simulink model "gm_broadwayIPC_2024b"  (R2024b)
settings: Solver=FixedStepDiscrete  StartTime=0.0  StopTime=2  RelTol=1e-3
undefined symbols (not defined in the file or in its folder): gray
libraries: hdlsllib x28, visionhdlio x6, visionsources x2
Description:
  | Sobel Edge Detection Using the MATLAB(R) Function Block
  | This example shows how to use HDL Coder(TM) to check,
  | generate, and verify HDL code for a Sobel Edge Detection
  | block built using the MATLAB Function block.
settings Model: Creator=The MathWorks, Inc.  LastModifiedBy=Chris
settings SolverCC: AlgebraicLoopSolver=TrustRegion
settings DataIOCC: LimitDataPoints=on  SaveFormat=Array  SignalLogging=off  ReturnWorkspaceOutputs=off
settings OptimizationCC: BlockReduction=off  ConditionallyExecuteInputs=off  DefaultParameterBehavior=Inlined  ExpressionDepthLimit=2147483647  InitFltsAndDblsToZero=on  EfficientMapNaN2IntZero=off  LifeSpan=inf
settings DebuggingCC: AlgebraicLoopMsg=error  SaveWithParameterizedLinksMsg=none  UnderspecifiedInitializationDetection=Classic  MergeDetectMultiDrivingBlocksExec=none  SignalResolutionControl=TryResolveAllWithWarning  InheritedTsInSrcMsg=none  MultiTaskDSMMsg=warning  MultiTaskCondExecSysMsg=none  SingleTaskRateTransMsg=error  IntegerOverflowMsg=none  ParameterPrecisionLossMsg=none  FcnCallInpInsideContextMsg=warning  UnconnectedInputMsg=warning  UnconnectedOutputMsg=warning  UnconnectedLineMsg=warning  AllowSymbolicDim=off  StateNameClashWarn=warning  StrictBusMsg=ErrorOnBusTreatedAsVector  SFUnexpectedBacktrackingDiag=warning  SFNoUnconditionalDefaultTransitionDiag=warning  SFExecutionAtInitializationDiag=none  IntegerSaturationMsg=none  ArithmeticOperatorsInVariantConditions=warning
settings HardwareCC: ProdBitPerPointer=32  ProdBitPerSizeT=32  ProdBitPerPtrDiffT=32  ProdLargestAtomicFloat=None  ProdIntDivRoundTo=Undefined  ProdEndianess=Unspecified  ProdWordSize=32  ProdHWDeviceType=ASIC/FPGA  TargetHWDeviceType=32-bit Generic  ProdEqTarget=off
settings ModelReferenceCC: EnableRefExpFcnMdlSchedulingChecks=on  PropagateSignalLabelsOutOfModel=off
settings SFSimCC: SimUseLocalCustomCode=off  CustomCodeUndefinedFunction=UseInterfaceOnly
settings RTWCC: RTWUseLocalCustomCode=off  GPUComputeCapability=3.5  DLArmComputeVersion=19.05
settings CodeAppCC: StateflowObjectComments=on
settings GRTTargetCC: TargetFcnLib=ansi_tfl_tmw.mat  TargetLangStandard=C89/C90 (ANSI)  CombineOutputUpdateFcns=off  GRTInterface=on
settings ConfigComp: CovMetricSettings=dw  CovSaveCumulativeToWorkspaceVar=on  CovSaveSingleToWorkspaceVar=on  CovExternalEMLEnable=off

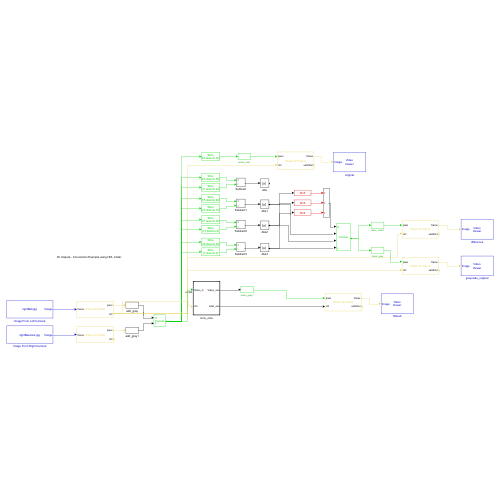
[thumbnail: Simulink's stored preview of the top-level diagram]
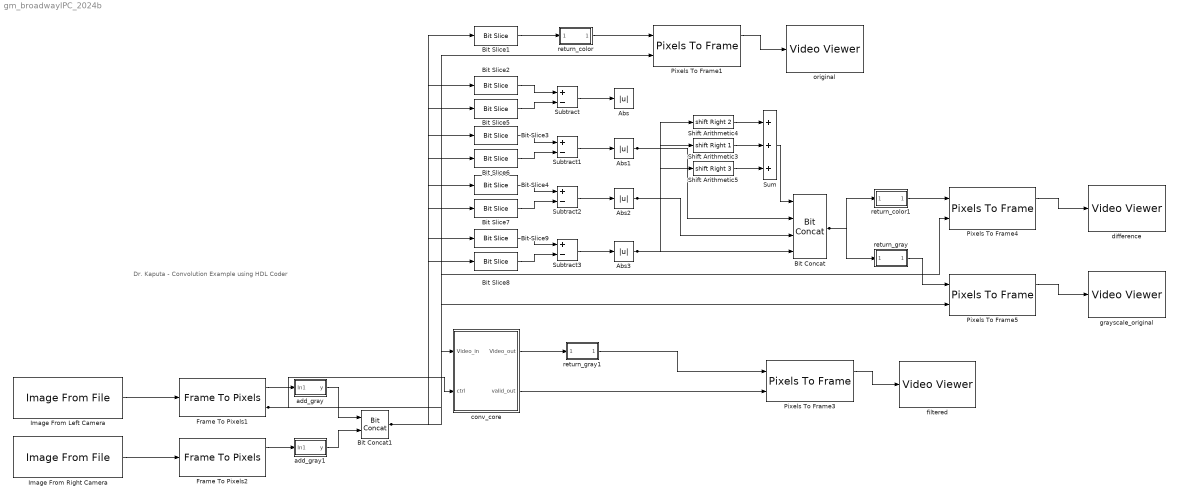
== system gm_broadwayIPC_2024b ==
  note: Dr. Kaputa - Convolution Example using HDL Coder
  Abs{,1..3} (4 alike) : Abs  OutDataTypeStr=uint8
  Bit Concat : hdlsllib/Logic and Bit Operations/Bit Concat  numInputs=4
  Bit Concat1 : hdlsllib/Logic and Bit Operations/Bit Concat  numInputs=2
  Bit Slice1 : hdlsllib/Logic and Bit Operations/Bit Slice  lidx=63  ridx=32
  Bit Slice2 : hdlsllib/Logic and Bit Operations/Bit Slice  lidx=63  ridx=56
  Bit Slice3 : hdlsllib/Logic and Bit Operations/Bit Slice  lidx=55  ridx=48
  Bit Slice4 : hdlsllib/Logic and Bit Operations/Bit Slice  lidx=47  ridx=40
  Bit Slice5 : hdlsllib/Logic and Bit Operations/Bit Slice  lidx=31  ridx=24
  Bit Slice6 : hdlsllib/Logic and Bit Operations/Bit Slice  lidx=23  ridx=16
  Bit Slice7 : hdlsllib/Logic and Bit Operations/Bit Slice  lidx=15  ridx=8
  Bit Slice8 : hdlsllib/Logic and Bit Operations/Bit Slice  lidx=7  ridx=0
  Bit Slice9 : hdlsllib/Logic and Bit Operations/Bit Slice  lidx=39  ridx=32
  Frame To Pixels1 : visionhdlio/Frame To Pixels  NumComponents=3  NumPixels=1  VideoFormat=Custom  ActivePixelsPerLine=R  ActiveVideoLines=C  TotalPixelsPerLine=R  TotalVideoLines=C  StartingActiveLine=1  FrontPorch=0  SampleTime=0  VideoFormatCache=Custom  ActivePixelsPerLineCache=R  ActiveVideoLinesCache=C  TotalPixelsPerLineCache=R  TotalVideoLinesCache=C  StartingActiveLineCache=1  FrontPorchCache=0
  Frame To Pixels2 : visionhdlio/Frame To Pixels  NumComponents=3  NumPixels=1  VideoFormat=Custom  ActivePixelsPerLine=R  ActiveVideoLines=C  TotalPixelsPerLine=R  TotalVideoLines=C  StartingActiveLine=1  FrontPorch=0  SampleTime=0  VideoFormatCache=Custom  ActivePixelsPerLineCache=R  ActiveVideoLinesCache=C  TotalPixelsPerLineCache=R  TotalVideoLinesCache=C  StartingActiveLineCache=1  FrontPorchCache=0
  Image From Left Camera : visionsources/Image From File  Tag=vipblks_nd  FileName=C:\Users\Chris\Documents\Repos\WiiSports\TennisTracker\BoradwaySimulink\rightBall.jpg  Ts=1  imagePorts=One multidimensional signal  OutPortLabels=R|G|B  ImageDataType=Inherit from input image  sdImageDataType=uint(8)  Signed=on  WordLength=16  FractionLengthMode=User-defined  FractionLength=15
  Image From Right Camera : visionsources/Image From File  Tag=vipblks_nd  FileName=C:\Users\Chris\Documents\Repos\WiiSports\TennisTracker\BoradwaySimulink\rightBaseline.jpg  Ts=1  imagePorts=One multidimensional signal  OutPortLabels=R|G|B  ImageDataType=Inherit from input image  sdImageDataType=uint(8)  Signed=on  WordLength=16  FractionLengthMode=User-defined  FractionLength=15
  Pixels To Frame1 : visionhdlio/Pixels To Frame  NumComponents=3  NumPixels=1  VideoFormat=Custom  ActivePixelsPerLine=R  ActiveVideoLines=C  TotalPixelsPerLine=R  TotalVideoLines=C  VideoFormatCache=Custom  ActivePixelsPerLineCache=R  ActiveVideoLinesCache=C  TotalPixelsPerLineCache=R  TotalVideoLinesCache=C
  Pixels To Frame3 : visionhdlio/Pixels To Frame  NumComponents=1  NumPixels=1  VideoFormat=Custom  ActivePixelsPerLine=R  ActiveVideoLines=C  TotalPixelsPerLine=R  TotalVideoLines=C  VideoFormatCache=Custom  ActivePixelsPerLineCache=R  ActiveVideoLinesCache=C  TotalPixelsPerLineCache=R  TotalVideoLinesCache=C
  Pixels To Frame4 : visionhdlio/Pixels To Frame  NumComponents=3  NumPixels=1  VideoFormat=Custom  ActivePixelsPerLine=R  ActiveVideoLines=C  TotalPixelsPerLine=R  TotalVideoLines=C  VideoFormatCache=Custom  ActivePixelsPerLineCache=R  ActiveVideoLinesCache=C  TotalPixelsPerLineCache=R  TotalVideoLinesCache=C
  Pixels To Frame5 : visionhdlio/Pixels To Frame  NumComponents=1  NumPixels=1  VideoFormat=Custom  ActivePixelsPerLine=R  ActiveVideoLines=C  TotalPixelsPerLine=R  TotalVideoLines=C  VideoFormatCache=Custom  ActivePixelsPerLineCache=R  ActiveVideoLinesCache=C  TotalPixelsPerLineCache=R  TotalVideoLinesCache=C
  Shift Arithmetic3 : ArithShift  BitShiftNumber=1  BitShiftDirection=Right
  Shift Arithmetic4 : ArithShift  BitShiftNumber=2  BitShiftDirection=Right
  Shift Arithmetic5 : ArithShift  BitShiftNumber=3  BitShiftDirection=Right
  Subtract{,1..3} (4 alike) : Sum  Inputs=+-
  Sum : Sum  Inputs=+++  OutDataTypeStr=uint8
  add_gray : Subsystem
  add_gray1 : Subsystem
  conv_core : Subsystem  TreatAsAtomicUnit=on
  difference : VideoViewer  FigPos=[994 1078 927 429]
  filtered : VideoViewer  colormapValue=gray(256)  FigPos=[66 1078 927 429]
  grayscale_original : VideoViewer  FigPos=[65 538 927 429]
  original : VideoViewer  FigPos=[995 538 927 429]
  return_color : Subsystem
  return_color1 : Subsystem
  return_gray : Subsystem
  return_gray1 : Subsystem
  wires:
  return_gray1/1(RGBVector) -> Pixels To Frame3/1
  conv_core/1(Video_out) -> return_gray1/1(RGB)
  Bit Concat/1 -> return_color1/1(RGB), return_gray/1(RGB)
  Sum/1 -> Bit Concat/1
  Abs1/1 -> Bit Concat/2, Shift Arithmetic4/1
  Abs2/1 -> Bit Concat/3, Shift Arithmetic3/1
  Abs3/1 -> Bit Concat/4, Shift Arithmetic5/1
  Shift Arithmetic4/1 -> Sum/1
  Shift Arithmetic3/1 -> Sum/2
  Shift Arithmetic5/1 -> Sum/3
  return_gray/1(RGBVector) -> Pixels To Frame5/1
  Pixels To Frame5/1 -> grayscale_original/1
  Bit Slice8/1 -> Subtract3/2
  Bit Slice9/1 -> Subtract3/1
  Bit Slice7/1 -> Subtract2/2
  Bit Slice4/1 -> Subtract2/1
  Bit Slice6/1 -> Subtract1/2
  Bit Slice3/1 -> Subtract1/1
  Bit Slice5/1 -> Subtract/2
  Bit Slice2/1 -> Subtract/1
  Subtract3/1 -> Abs3/1
  Subtract2/1 -> Abs2/1
  Subtract1/1 -> Abs1/1
  return_color1/1(RGBVector) -> Pixels To Frame4/1
  Subtract/1 -> Abs/1
  Pixels To Frame4/1 -> difference/1
  Bit Slice1/1 -> return_color/1(RGB)
  add_gray1/1(y) -> Bit Concat1/2
  add_gray/1(y) -> Bit Concat1/1
  Frame To Pixels2/1 -> add_gray1/1(In1)
  Frame To Pixels1/2 -> conv_core/2(ctrl), Pixels To Frame4/2, Pixels To Frame5/2, Pixels To Frame1/2
  Image From Right Camera/1 -> Frame To Pixels2/1
  Bit Concat1/1 -> conv_core/1(Video_in), Bit Slice5/1, Bit Slice3/1, Bit Slice6/1, Bit Slice4/1, Bit Slice7/1, Bit Slice9/1, Bit Slice8/1, Bit Slice2/1, Bit Slice1/1
  conv_core/2(valid_out) -> Pixels To Frame3/2
  Pixels To Frame3/1 -> filtered/1
  Frame To Pixels1/1 -> add_gray/1(In1)
  return_color/1(RGBVector) -> Pixels To Frame1/1
  Pixels To Frame1/1 -> original/1
  Image From Left Camera/1 -> Frame To Pixels1/1

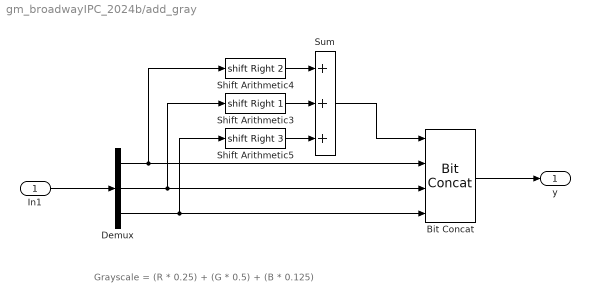
== system gm_broadwayIPC_2024b/add_gray ==
  note: Grayscale = (R * 0.25) + (G * 0.5) + (B * 0.125)
  In1 : Inport
  Bit Concat : hdlsllib/Logic and Bit Operations/Bit Concat  numInputs=4
  Demux : Demux  Outputs=3
  Shift Arithmetic3 : ArithShift  BitShiftNumber=1  BitShiftDirection=Right
  Shift Arithmetic4 : ArithShift  BitShiftNumber=2  BitShiftDirection=Right
  Shift Arithmetic5 : ArithShift  BitShiftNumber=3  BitShiftDirection=Right
  Sum : Sum  Inputs=+++  OutDataTypeStr=uint8
  y : Outport
  wires:
  Shift Arithmetic5/1 -> Sum/3
  Shift Arithmetic3/1 -> Sum/2
  Shift Arithmetic4/1 -> Sum/1
  Sum/1 -> Bit Concat/1
  Demux/3 -> Bit Concat/4, Shift Arithmetic5/1
  Demux/1 -> Bit Concat/2, Shift Arithmetic4/1
  Demux/2 -> Bit Concat/3, Shift Arithmetic3/1
  In1/1 -> Demux/1
  Bit Concat/1 -> y/1

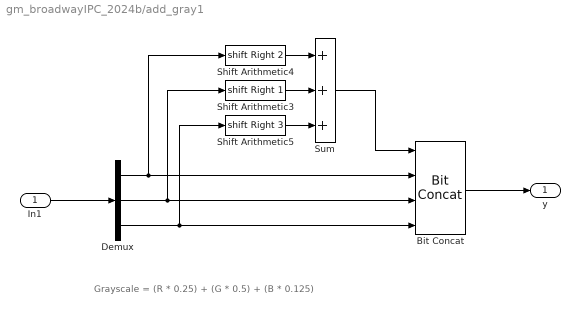
== system gm_broadwayIPC_2024b/add_gray1 ==
  note: Grayscale = (R * 0.25) + (G * 0.5) + (B * 0.125)
  In1 : Inport
  Bit Concat : hdlsllib/Logic and Bit Operations/Bit Concat  numInputs=4
  Demux : Demux  Outputs=3
  Shift Arithmetic3 : ArithShift  BitShiftNumber=1  BitShiftDirection=Right
  Shift Arithmetic4 : ArithShift  BitShiftNumber=2  BitShiftDirection=Right
  Shift Arithmetic5 : ArithShift  BitShiftNumber=3  BitShiftDirection=Right
  Sum : Sum  Inputs=+++  OutDataTypeStr=uint8
  y : Outport
  wires:
  Sum/1 -> Bit Concat/1
  Shift Arithmetic5/1 -> Sum/3
  Shift Arithmetic3/1 -> Sum/2
  Shift Arithmetic4/1 -> Sum/1
  Demux/3 -> Bit Concat/4, Shift Arithmetic5/1
  Demux/1 -> Bit Concat/2, Shift Arithmetic4/1
  Demux/2 -> Bit Concat/3, Shift Arithmetic3/1
  In1/1 -> Demux/1
  Bit Concat/1 -> y/1

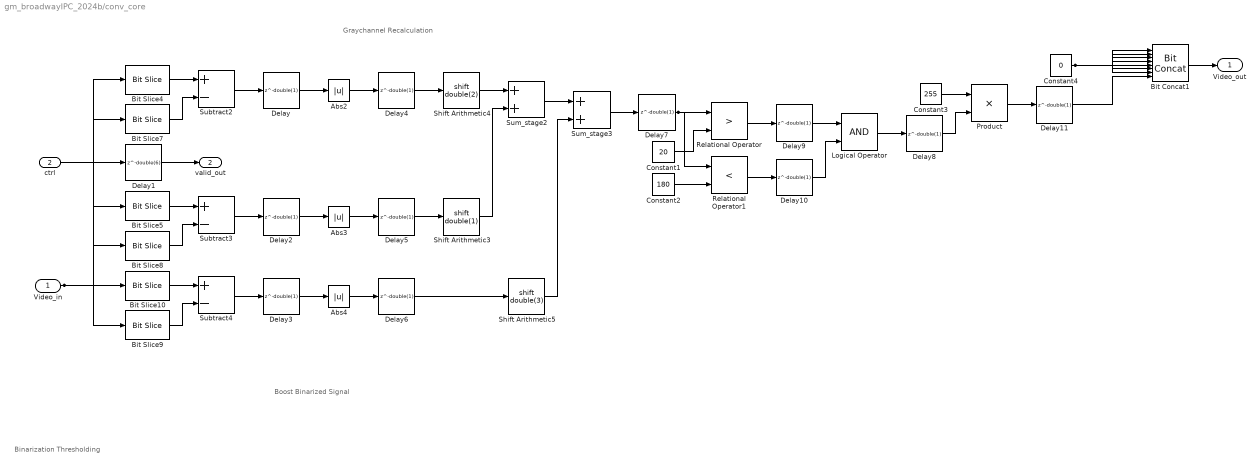
== system gm_broadwayIPC_2024b/conv_core ==
  note: Boost Binarized Signal
  note: Binarization Thresholding
  note: Graychannel Recalculation
  Video_in : Inport  OutDataTypeStr=fixdt(0, 64, 0)  PortDimensions=1  SampleTime=2.77039007092199e-06
  ctrl : Inport  Port=2
  Abs2 : Abs  SampleTime=2.77039007092199e-06  OutDataTypeStr=uint8  SaturateOnIntegerOverflow=off
  Abs3 : Abs  SampleTime=2.77039007092199e-06  OutDataTypeStr=uint8  SaturateOnIntegerOverflow=off
  Abs4 : Abs  SampleTime=2.77039007092199e-06  OutDataTypeStr=uint8  SaturateOnIntegerOverflow=off
  Bit Concat1 : hdlsllib/Logic and Bit Operations/Bit Concat  numInputs=8
  Bit Slice10 : hdlsllib/Logic and Bit Operations/Bit Slice  lidx=double(39)  ridx=double(32)
  Bit Slice4 : hdlsllib/Logic and Bit Operations/Bit Slice  lidx=double(55)  ridx=double(48)
  Bit Slice5 : hdlsllib/Logic and Bit Operations/Bit Slice  lidx=double(47)  ridx=double(40)
  Bit Slice7 : hdlsllib/Logic and Bit Operations/Bit Slice  lidx=double(23)  ridx=double(16)
  Bit Slice8 : hdlsllib/Logic and Bit Operations/Bit Slice  lidx=double(15)  ridx=double(8)
  Bit Slice9 : hdlsllib/Logic and Bit Operations/Bit Slice  lidx=double(7)  ridx=double(0)
  Constant1 : Constant  Value=20  OutDataTypeStr=uint8  SampleTime=2.77039007092199e-06
  Constant2 : Constant  Value=180  OutDataTypeStr=uint8  SampleTime=2.77039007092199e-06
  Constant3 : Constant  Value=255  OutDataTypeStr=uint8  SampleTime=2.77039007092199e-06
  Constant4 : Constant  Value=0  OutDataTypeStr=uint8  SampleTime=2.77039007092199e-06
  Delay{,2..11} (11 alike) : Delay  DelayLength=double(1)  InitialCondition=0  SampleTime=2.77039007092199e-06
  Delay1 : Delay  DelayLength=double(6)  InitialCondition=0  SampleTime=2.77039007092199e-06
  Logical Operator : Logic  AllPortsSameDT=off  OutDataTypeStr=boolean  SampleTime=2.77039007092199e-06
  Product : Product  Inputs=**  OutDataTypeStr=uint8  SampleTime=2.77039007092199e-06
  Relational Operator : RelationalOperator  Operator=>  OutDataTypeStr=boolean  SampleTime=2.77039007092199e-06  InputSameDT=off
  Relational Operator1 : RelationalOperator  Operator=<  OutDataTypeStr=boolean  SampleTime=2.77039007092199e-06  InputSameDT=off
  Shift Arithmetic3 : ArithShift  BitShiftNumber=double(1)  BinPtShiftNumber=double(0)
  Shift Arithmetic4 : ArithShift  BitShiftNumber=double(2)  BinPtShiftNumber=double(0)
  Shift Arithmetic5 : ArithShift  BitShiftNumber=double(3)  BinPtShiftNumber=double(0)
  Subtract2 : Sum  Inputs=+-  OutDataTypeStr=fixdt(1, 9, 0)  AccumDataTypeStr=fixdt(1, 9, 0)  SampleTime=2.77039007092199e-06
  Subtract3 : Sum  Inputs=+-  OutDataTypeStr=fixdt(1, 9, 0)  AccumDataTypeStr=fixdt(1, 9, 0)  SampleTime=2.77039007092199e-06
  Subtract4 : Sum  Inputs=+-  OutDataTypeStr=fixdt(1, 9, 0)  AccumDataTypeStr=fixdt(1, 9, 0)  SampleTime=2.77039007092199e-06
  Sum_stage2 : Sum  OutDataTypeStr=fixdt(0, 9, 0)  AccumDataTypeStr=uint8  SampleTime=2.77039007092199e-06
  Sum_stage3 : Sum  OutDataTypeStr=uint8  AccumDataTypeStr=uint8  SampleTime=2.77039007092199e-06
  Video_out : Outport  SampleTime=2.77039007092199e-06  VectorParamsAs1DForOutWhenUnconnected=off
  valid_out : Outport  Port=2  VectorParamsAs1DForOutWhenUnconnected=off
  wires:
  Delay3/1 -> Abs4/1
  ctrl/1 -> Delay1/1
  Delay11/1 -> Bit Concat1/8
  Bit Slice10/1 -> Subtract4/1
  Video_in/1 -> Bit Slice9/1, Bit Slice5/1, Bit Slice7/1, Bit Slice4/1, Bit Slice8/1, Bit Slice10/1
  Delay1/1 -> valid_out/1
  Shift Arithmetic3/1 -> Sum_stage2/2
  Bit Slice4/1 -> Subtract2/1
  Bit Slice7/1 -> Subtract2/2
  Sum_stage3/1 -> Delay7/1
  Bit Slice5/1 -> Subtract3/1
  Bit Slice8/1 -> Subtract3/2
  Bit Slice9/1 -> Subtract4/2
  Subtract2/1 -> Delay/1
  Abs4/1 -> Delay6/1
  Subtract3/1 -> Delay2/1
  Subtract4/1 -> Delay3/1
  Delay/1 -> Abs2/1
  Delay2/1 -> Abs3/1
  Abs2/1 -> Delay4/1
  Abs3/1 -> Delay5/1
  Delay4/1 -> Shift Arithmetic4/1
  Delay5/1 -> Shift Arithmetic3/1
  Logical Operator/1 -> Delay8/1
  Delay6/1 -> Shift Arithmetic5/1
  Shift Arithmetic4/1 -> Sum_stage2/1
  Sum_stage2/1 -> Sum_stage3/1
  Shift Arithmetic5/1 -> Sum_stage3/2
  Delay7/1 -> Relational Operator1/1, Relational Operator/1
  Constant1/1 -> Relational Operator/2
  Constant2/1 -> Relational Operator1/2
  Relational Operator/1 -> Delay9/1
  Delay9/1 -> Logical Operator/1
  Relational Operator1/1 -> Delay10/1
  Delay10/1 -> Logical Operator/2
  Constant3/1 -> Product/1
  Delay8/1 -> Product/2
  Product/1 -> Delay11/1
  Constant4/1 -> Bit Concat1/6, Bit Concat1/5, Bit Concat1/3, Bit Concat1/4, Bit Concat1/2, Bit Concat1/7, Bit Concat1/1
  Bit Concat1/1 -> Video_out/1

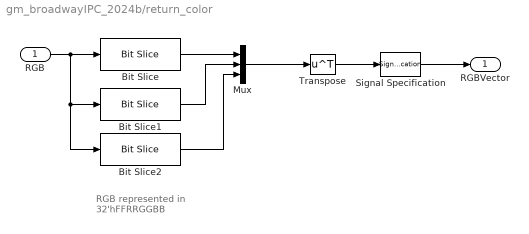
== system gm_broadwayIPC_2024b/return_color ==
  note: RGB represented in
      | 32'hFFRRGGBB
  RGB : Inport
  Bit Slice : hdlsllib/Logic and Bit Operations/Bit Slice  lidx=23  ridx=16
  Bit Slice1 : hdlsllib/Logic and Bit Operations/Bit Slice  lidx=15  ridx=8
  Bit Slice2 : hdlsllib/Logic and Bit Operations/Bit Slice  lidx=7  ridx=0
  Mux : Mux  Inputs=3
  Signal Specification : SignalSpecification
  Transpose : Math  Operator=transpose  SignedPower=on
  RGBVector : Outport  VectorParamsAs1DForOutWhenUnconnected=off
  wires:
  Mux/1 -> Transpose/1
  Bit Slice/1 -> Mux/1
  Bit Slice2/1 -> Mux/3
  Bit Slice1/1 -> Mux/2
  RGB/1 -> Bit Slice2/1, Bit Slice1/1, Bit Slice/1
  Transpose/1 -> Signal Specification/1
  Signal Specification/1 -> RGBVector/1

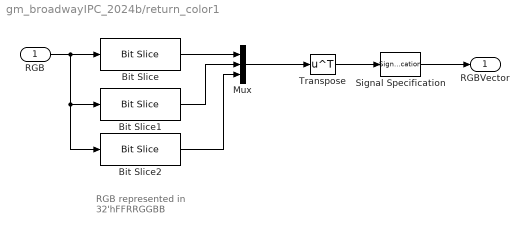
== system gm_broadwayIPC_2024b/return_color1 ==
  note: RGB represented in
      | 32'hFFRRGGBB
  RGB : Inport
  Bit Slice : hdlsllib/Logic and Bit Operations/Bit Slice  lidx=23  ridx=16
  Bit Slice1 : hdlsllib/Logic and Bit Operations/Bit Slice  lidx=15  ridx=8
  Bit Slice2 : hdlsllib/Logic and Bit Operations/Bit Slice  lidx=7  ridx=0
  Mux : Mux  Inputs=3
  Signal Specification : SignalSpecification
  Transpose : Math  Operator=transpose  SignedPower=on
  RGBVector : Outport  VectorParamsAs1DForOutWhenUnconnected=off
  wires:
  Mux/1 -> Transpose/1
  Bit Slice/1 -> Mux/1
  Bit Slice2/1 -> Mux/3
  Bit Slice1/1 -> Mux/2
  RGB/1 -> Bit Slice2/1, Bit Slice1/1, Bit Slice/1
  Transpose/1 -> Signal Specification/1
  Signal Specification/1 -> RGBVector/1

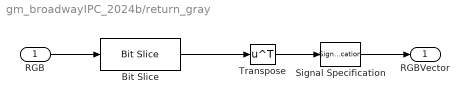
== system gm_broadwayIPC_2024b/return_gray ==
  RGB : Inport
  Bit Slice : hdlsllib/Logic and Bit Operations/Bit Slice  lidx=31  ridx=24
  Signal Specification : SignalSpecification
  Transpose : Math  Operator=transpose  SignedPower=on
  RGBVector : Outport  VectorParamsAs1DForOutWhenUnconnected=off
  wires:
  Bit Slice/1 -> Transpose/1
  Signal Specification/1 -> RGBVector/1
  Transpose/1 -> Signal Specification/1
  RGB/1 -> Bit Slice/1

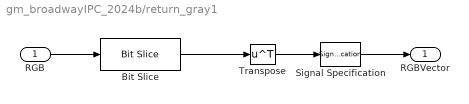
== system gm_broadwayIPC_2024b/return_gray1 ==
  RGB : Inport
  Bit Slice : hdlsllib/Logic and Bit Operations/Bit Slice  lidx=7  ridx=0
  Signal Specification : SignalSpecification
  Transpose : Math  Operator=transpose  SignedPower=on
  RGBVector : Outport  VectorParamsAs1DForOutWhenUnconnected=off
  wires:
  Bit Slice/1 -> Transpose/1
  Signal Specification/1 -> RGBVector/1
  Transpose/1 -> Signal Specification/1
  RGB/1 -> Bit Slice/1
